simulink model "tiny"  (Simulink 7.6)
settings: Solver=FixedStepDiscrete  StartTime=0.0  StopTime=10.0  FixedStep=0.2  RelTol=1e-3
settings Model: Creator=developer  LastModifiedBy=developer
settings DebuggingCC: StrictBusMsg=ErrorOnBusTreatedAsVector  NonBusSignalsTreatedAsBus=error

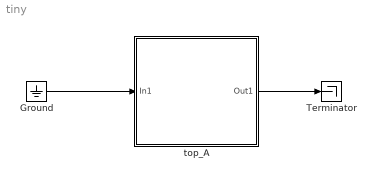
== system tiny ==
  Ground : Ground
  Terminator : Terminator
  top_A : Subsystem  TreatAsAtomicUnit=on
  wires:
  top_A/1(Out1) -> Terminator/1
  Ground/1 -> top_A/1(In1)

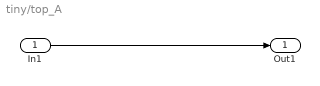
== system tiny/top_A ==
  In1 : Inport
  Out1 : Outport
  wires:
  In1/1 -> Out1/1
